simulink model "msg2data"  (R2016a)
settings: Solver=VariableStepAuto  StartTime=0.0  StopTime=inf  RelTol=1e-3
undefined symbols (not defined in the file): Ae, Be, Ce, De, Tsample
libraries: etargetslib x2, dspnetwork x2, utility x1
settings Model: Creator=Florian  LastModifiedBy=Florian

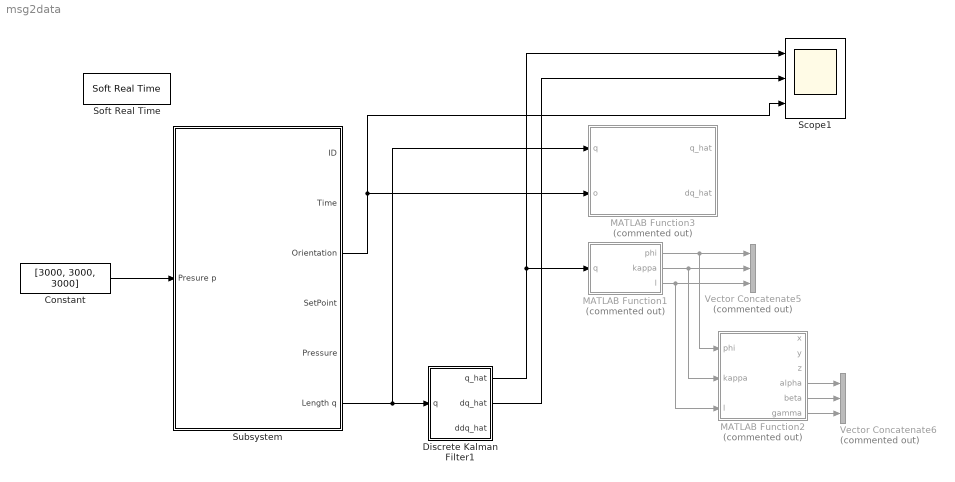
== system msg2data ==
  Constant : Constant  Value=[3000, 3000, 3000]
  Discrete Kalman Filter1 : MATLAB Function  TreatAsAtomicUnit=on  SystemSampleTime=Tsample
  MATLAB Function1 : MATLAB Function  Commented=on  TreatAsAtomicUnit=on
  MATLAB Function2 : MATLAB Function  Commented=on  TreatAsAtomicUnit=on
  MATLAB Function3 : MATLAB Function  Commented=on  TreatAsAtomicUnit=on
  Scope1 : Scope  NumInputPorts=3
  Soft Real Time : utility/Soft Real Time  x=1
  Subsystem : Subsystem
      mask Display: image('C:\Users\Florian\Documents\Uni\IDP\DVD\Pictures\contibot1seg.JPG');
  Vector Concatenate5 : Concatenate  Commented=on  NumInputs=3
  Vector Concatenate6 : Concatenate  Commented=on  NumInputs=3
  wires:
  MATLAB Function1/1(phi) -> Vector Concatenate5/1, MATLAB Function2/1(phi)
  MATLAB Function1/2(kappa) -> Vector Concatenate5/2, MATLAB Function2/2(kappa)
  MATLAB Function1/3(l) -> Vector Concatenate5/3, MATLAB Function2/3(l)
  Discrete Kalman Filter1/1(q_hat) -> Scope1/1, MATLAB Function1/1(q)
  MATLAB Function2/6(gamma) -> Vector Concatenate6/3
  MATLAB Function2/5(beta) -> Vector Concatenate6/2
  MATLAB Function2/4(alpha) -> Vector Concatenate6/1
  Subsystem/6(Length q) -> MATLAB Function3/1(q), Discrete Kalman Filter1/1(q)
  Constant/1 -> Subsystem/1(Presure p)
  Subsystem/3(Orientation) -> Scope1/3, MATLAB Function3/2(o)
  Discrete Kalman Filter1/2(dq_hat) -> Scope1/2

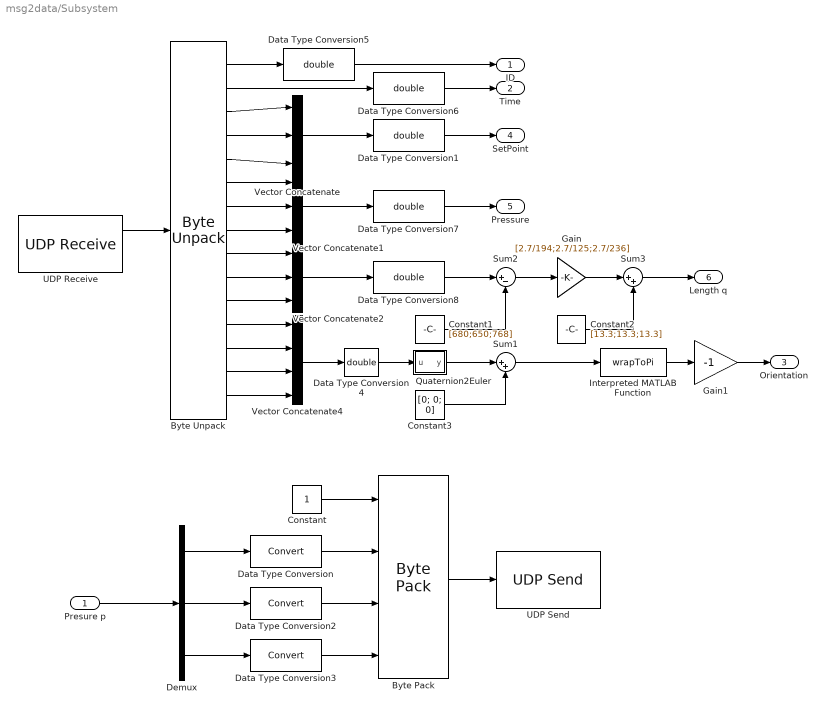
== system msg2data/Subsystem ==
  Presure p : Inport
  Byte Pack : etargetslib/Byte Pack  datatypes={'uint32', 'uint32', 'uint32', 'uint32'}  byteAlign=1
  Byte Unpack : etargetslib/Byte Unpack  dimensions={[1],[1],[1],[1],[1],[1],[1],[1],[1],[1],[1],[1],[1],[1],[1]}  datatypes={'uint32', 'uint32', 'uint32', 'uint32', 'uint32', 'uint32', 'uint32', 'uint32', 'single', 'single', 'single', 'single', 'single', 'single', 'single'}  byteAlign=1
  Constant : Constant  OutDataTypeStr=uint32
  Constant1 : Constant  Value=[680;650;768]  OutDataTypeStr=uint32
  Constant2 : Constant  Value=[13.3;13.3;13.3]  OutDataTypeStr=uint32
  Constant3 : Constant  Value=[0; 0; 0]  OutDataTypeStr=uint32
  Data Type Conversion : DataTypeConversion
  Data Type Conversion{1,4..8} (6 alike) : DataTypeConversion  OutDataTypeStr=double
  Data Type Conversion2 : DataTypeConversion
  Data Type Conversion3 : DataTypeConversion
  Demux : Demux  Outputs=3
  Gain : Gain  Gain=[2.7/194;2.7/125;2.7/236]
  Gain1 : Gain  Gain=-1
  Interpreted MATLAB Function : MATLABFcn  MATLABFcn=wrapToPi
  Quaternion2Euler : MATLAB Function  TreatAsAtomicUnit=on
  Sum1 : Sum  Inputs=|++
  Sum2 : Sum  Inputs=|+-
  Sum3 : Sum  Inputs=|++
  UDP Receive : dspnetwork/UDP Receive  localURL='0.0.0.0'  localPort=25000  remoteURL='0.0.0.0'  remotePort=-1  recvBufferSize=256  dims=15*4  signalDatatype=uint8  isVarSize=off  showBlockingTime=on  blockingTime=0  sampletime=0.01  blockPlatform=HOST
  UDP Send : dspnetwork/UDP Send  remoteURL='127.0.0.1'  remotePort=12345  localURL='0.0.0.0'  localPortSource=Specify via dialog  localPort=25000  sampletime=-1  blockPlatform=HOST  separateLengthPort=0
  Vector Concatenate : Concatenate  NumInputs=3
  Vector Concatenate1 : Concatenate  NumInputs=3
  Vector Concatenate2 : Concatenate  NumInputs=3
  Vector Concatenate4 : Concatenate  NumInputs=4
  ID : Outport
  Time : Outport  Port=2
  Orientation : Outport  Port=3
  SetPoint : Outport  Port=4
  Pressure : Outport  Port=5
  Length q : Outport  Port=6
  wires:
  Gain1/1 -> Orientation/1
  Constant3/1 -> Sum1/2
  Sum1/1 -> Interpreted MATLAB Function/1
  Interpreted MATLAB Function/1 -> Gain1/1
  Byte Unpack/9 -> Vector Concatenate2/1
  Constant/1 -> Byte Pack/1
  Vector Concatenate/1 -> Data Type Conversion1/1
  Byte Unpack/6 -> Vector Concatenate1/1
  Sum2/1 -> Gain/1
  Gain/1 -> Sum3/1
  Byte Unpack/4 -> Vector Concatenate/2
  Byte Pack/1 -> UDP Send/1
  Byte Unpack/3 -> Vector Concatenate/1
  Byte Unpack/12 -> Vector Concatenate4/1
  Byte Unpack/5 -> Vector Concatenate/3
  Byte Unpack/13 -> Vector Concatenate4/2
  Constant2/1 -> Sum3/2
  Byte Unpack/14 -> Vector Concatenate4/3
  UDP Receive/1 -> Byte Unpack/1
  Byte Unpack/10 -> Vector Concatenate2/2
  Byte Unpack/7 -> Vector Concatenate1/2
  Byte Unpack/8 -> Vector Concatenate1/3
  Byte Unpack/11 -> Vector Concatenate2/3
  Sum3/1 -> Length q/1
  Byte Unpack/15 -> Vector Concatenate4/4
  Constant1/1 -> Sum2/2
  Quaternion2Euler/1(y) -> Sum1/1
  Vector Concatenate2/1 -> Data Type Conversion8/1
  Data Type Conversion1/1 -> SetPoint/1
  Byte Unpack/1 -> Data Type Conversion5/1
  Data Type Conversion5/1 -> ID/1
  Data Type Conversion6/1 -> Time/1
  Byte Unpack/2 -> Data Type Conversion6/1
  Vector Concatenate1/1 -> Data Type Conversion7/1
  Data Type Conversion7/1 -> Pressure/1
  Data Type Conversion8/1 -> Sum2/1
  Demux/1 -> Data Type Conversion/1
  Demux/2 -> Data Type Conversion2/1
  Presure p/1 -> Demux/1
  Demux/3 -> Data Type Conversion3/1
  Vector Concatenate4/1 -> Data Type Conversion4/1
  Data Type Conversion4/1 -> Quaternion2Euler/1(u)
  Data Type Conversion/1 -> Byte Pack/2
  Data Type Conversion2/1 -> Byte Pack/3
  Data Type Conversion3/1 -> Byte Pack/4

== matlab function msg2data/MATLAB Function1 ==
  data: q input; phi output; kappa output; l output
function [phi, kappa, l] = fcn(q)
%#codegen
q = double(q / 100);
rB = 2/100;

if q(1) == q(2) && q(2) == q(3)
    phi = 0;
    kappa = 0;
    l = q(1);
else
    phi = atan2(sqrt(3)*(q(3)-q(2)), q(2)+q(3)-2*q(1));
    kappa = 2 * sqrt(q(1)^2 + q(2)^2 + q(3)^2 - q(1)*q(2) - q(2)*q(3) - q(3)*q(1)) / ((q(1)+q(2)+q(3))*rB);
    l = (q(1)+q(2)+q(3))/3;
end

== matlab function msg2data/Subsystem/Quaternion2Euler ==
  data: u input; y output
function y = fcn(u)
%#codegen
u = u / 1000;
y = zeros(3,1);

y(1) = atan2(2*(u(1)*u(2)+u(3)*u(4)),1-2*(u(2)*u(2)+u(3)*u(3)));

if abs(2*(u(1)*u(3)-u(4)*u(2))) > 1
    y(2) = 0;
else
    y(2) = asin(2*(u(1)*u(3)-u(4)*u(2)));
end
y(3) = atan2(2*(u(1)*u(4)+u(2)*u(3)),1-2*(u(3)*u(3)+u(4)*u(4)));

== matlab function msg2data/MATLAB Function2 ==
  data: phi input; x output; y output; z output; kappa input; l input; alpha output; beta output; gamma output
function [x, y, z, alpha, beta, gamma] = fcn(phi, kappa, l)
%#codegen
c_phi = cos(phi);
s_phi = sin(phi);
c_kl = cos(kappa*l);
s_kl = sin(kappa*l);

H = [c_phi^2*(c_kl-1)+1, s_phi*c_phi*(c_kl-1), c_phi*s_phi, c_phi*(1-c_kl)/kappa; ...
     c_phi*s_phi*(c_kl-1), c_phi^2*(c_kl-1)+c_kl, s_phi*s_kl, s_phi*(1-c_kl)/kappa; ...
     -c_phi*s_kl, -s_phi*s_kl, c_kl, s_kl/kappa; ...
     0, 0, 0, 1];
 
 x = H(1, 4);
 y = H(2, 4);
 z = H(3, 4);
 
 beta = atan2(-H(3, 1), sqrt(H(1,1)^2+H(2, 1)^2));
 if abs(beta) == pi/2
     alpha = 0;
     gamma = sign(beta) * atan2(H(1,2), H(2,2));
 else
     alpha = atan2(H(2,1), H(1,1));
     gamma = atan2(H(3,2), H(3,3));
 end

== matlab function msg2data/Discrete Kalman Filter1 ==
  data: Ae parameter; Be parameter; Ce parameter; De parameter; q input; q_hat output; dq_hat output; ddq_hat output
function [q_hat,dq_hat, ddq_hat] = fcn(Ae,Be,Ce,De,q)
%#codegen
persistent x
if isempty(x)
   x = zeros(3, length(q));%[0;0];
end
 
q_hat = zeros(size(q));
dq_hat = q_hat;
ddq_hat = dq_hat;

for i = 1:length(q)
x_pred = Ae * x(:, i) + Be * q(i);
hat = Ce * x(:, i) + De * q(i);
x(:, i) = x_pred;

y_hat = hat(1);
x_hat = hat(2:4,1);

q_hat(i) = x_hat(1);
dq_hat(i) = x_hat(2);
ddq_hat(i) = x_hat(3);
end

== matlab function msg2data/MATLAB Function3 ==
  data: q input; q_hat output; dq_hat output; o input
function [q_hat, dq_hat] = fcn(q, o)

q = q / 100;

%#codegen
persistent x P
if isempty(x)
   x = zeros(6, 1);%[0;0];
   P = eye(6);
end

T = 0.01;
F = [1 0 0  0 0 0;...
     0 1 0  0 0 0;...
     0 0 1  0 0 0;...
     T 0 0  1 0 0;...
     0 T 0  0 1 0;...
     0 0 T  0 0 1];
 
Q = 0.0001 * ones(6);
R = Q;
 
% Prediction:
x_pred = F * x;
P_pred = F * P * F' + Q; 

% Correction:
z = [q; o];
[alpha_pred, beta_pred, gamma_pred] = GetOrientation(x_pred(4:6));
z_pred = [x_pred(4:6); alpha_pred; beta_pred; gamma_pred];

y = z - z_pred;
H = [0 0 0  1 0 0;...
     0 0 0  0 1 0;...
     0 0 0  0 0 1;...
     0 0 0  dAlphadq(x_pred(4), x_pred(5), x_pred(6));...
     0 0 0  dBetadq(x_pred(4), x_pred(5), x_pred(6));...
     0 0 0  dGammadq(x_pred(4), x_pred(5), x_pred(6))];
S = H * P_pred * H' + R;
K = P_pred * H' * pinv(S);
x = x_pred + K * y;
P = (eye(size(H)) - K*H)*P_pred;

q_hat = x(4:6);
dq_hat = x(1:3);

end
